simulink model "PFC_V10"  (R2016b)
settings: Solver=FixedStepDiscrete  StartTime=0.0  StopTime=0.1  FixedStep=1e-7  RelTol=1e-3
libraries: powerlib x15, simulink x1
settings Model: Creator=a037702  LastModifiedBy=a037702

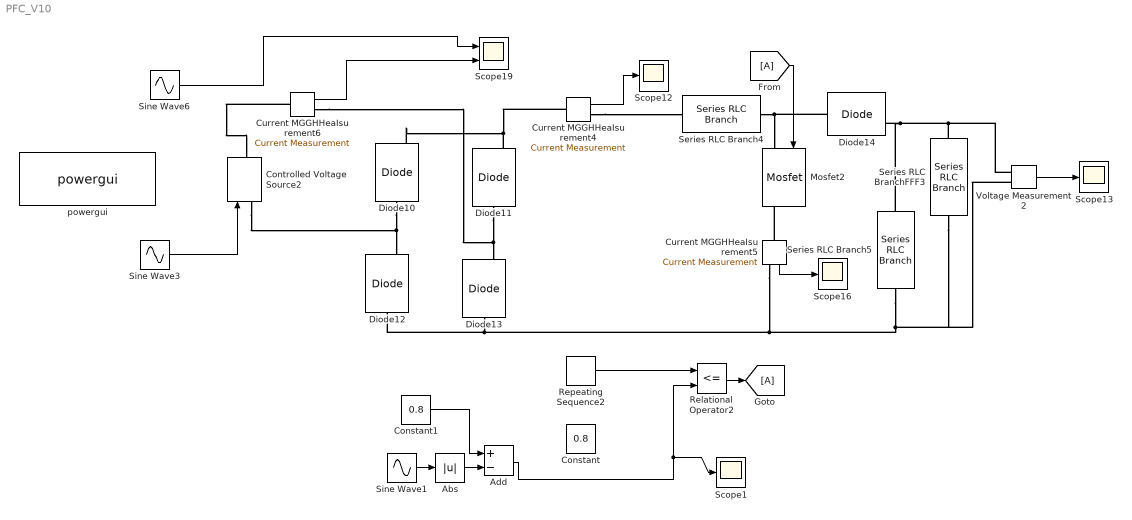
== system PFC_V10 ==
  Abs : Abs
  Add : Sum  Inputs=+-
  Constant : Constant  Value=0.8
  Constant1 : Constant  Value=0.8
  Controlled Voltage Source2 : powerlib/Electrical Sources/Controlled Voltage Source  Initialize=on  Source_Type=AC  Amplitude=0  Phase=0  Frequency=0  Measurements=None
  Current MGGHHeaIsurement4 : powerlib/Measurements/Current Measurement  PhasorSimulation=off  OutputType=Complex  PSBequivalent=0
  Current MGGHHeaIsurement5 : powerlib/Measurements/Current Measurement  PhasorSimulation=off  OutputType=Complex  PSBequivalent=0
  Current MGGHHeaIsurement6 : powerlib/Measurements/Current Measurement  PhasorSimulation=off  OutputType=Complex  PSBequivalent=0
  Diode{10..14} (5 alike) : powerlib/Power Electronics/Diode  Ron=0.001  Lon=0  Vf=0.8  IC=0  UseSnubber=off  Rs=500  Cs=250e-9  Measurements=on
  Mosfet2 : powerlib/Power Electronics/Mosfet  Ron=0.1  Lon=0  Rd=0.01  Vfd=0  IC=0  Rs=1e5  Cs=inf  Measurements=on
  Relational Operator2 : RelationalOperator  Operator=<=  OutDataTypeStr=boolean  RndMeth=Simplest
  Repeating Sequence2 : simulink/Sources/Repeating Sequence  rep_seq_t=[0 10e-6]  rep_seq_y=[0 1]
  Scope{1,12..13,16} (4 alike) : Scope
  Scope19 : Scope  NumInputPorts=2
  Series RLC Branch4 : powerlib/Elements/Series RLC Branch  LConnTagsString=__new0  RConnTagsString=__new0  BranchType=L  Resistance=1  Inductance=500e-6  SetiL0=on  InitialCurrent=0  Capacitance=1e-6  Setx0=off  InitialVoltage=0  Measurements=Branch current
  Series RLC Branch5 : powerlib/Elements/Series RLC Branch  LConnTagsString=__new0  RConnTagsString=__new0  BranchType=R  Resistance=100  Inductance=500e-6  SetiL0=on  InitialCurrent=0  Capacitance=100e-6  Setx0=on  InitialVoltage=0  Measurements=Branch current
  Series RLC BranchFFF3 : powerlib/Elements/Series RLC Branch  LConnTagsString=__new0  RConnTagsString=__new0  BranchType=C  Resistance=1  Inductance=500e-6  SetiL0=on  InitialCurrent=0  Capacitance=100e-6  Setx0=on  InitialVoltage=0  Measurements=Branch current
  Sine Wave1 : Sin  Amplitude=0.3  Frequency=2*pi*50  SampleTime=0
  Sine Wave3 : Sin  Amplitude=320  Frequency=2*pi*50  SampleTime=0
  Sine Wave6 : Sin  Amplitude=20  Frequency=2*pi*50  SampleTime=0
  Voltage Measurement2 : powerlib/Measurements/Voltage Measurement  PhasorSimulation=off  OutputType=Complex  PSBequivalent=0
  powergui : powerlib/powergui  Priority=1  SimulationMode=Discrete  SolverType=Tustin/Backward Euler (TBE)  SampleTime=.1e-6  frequency=60  SPID=off  DisableSnubberDevices=off  DisableRonSwitches=off  DisableVfSwitches=off  SwTol=0  DisplayEquations=off  Interpol=off  ExternalGateDelay=off  methode=off  Ts=10  FunctionMessages=off  echomessages=off  HookPort=off  EnableUseOfTLC=off  x0status=blocks  frequencyindice=0  Pbase=100e6  ErrMax=1e-4  Iterations=50  UnitsV=kV  UnitsW=MW  buscounter=0  RestoreLinks=warning  ResistiveCurrentMeasurement=off  Frange=[0:2:500]  Ylog=off  Xlog=on  ShowGrid=off  save=off  variable=ZData  structure=0  ZoomFFT=off  StartTime=0.0  cycles=1  DisplayStyle=1  fundamental=60  FreqAxis=off  MaxFrequency=1000  frequencyindicesteady=1  RmsSteady=1  display=off
  wires:
  Sine Wave3/1 -> Controlled Voltage Source2/1
  Current MGGHHeaIsurement4/1 -> Scope12/1
  Voltage Measurement2/1 -> Scope13/1
  Current MGGHHeaIsurement5/1 -> Scope16/1
  Repeating Sequence2/1 -> Relational Operator2/1
  Current MGGHHeaIsurement6/1 -> Scope19/2
  Sine Wave6/1 -> Scope19/1
  Add/1 -> Scope1/1, Relational Operator2/2
  Relational Operator2/1 -> [A]
  [A] -> Mosfet2/1
  Sine Wave1/1 -> Abs/1
  Abs/1 -> Add/2
  Constant1/1 -> Add/1
  connections:
  Diode11/RConn1 -- Diode10/RConn1 -- Current MGGHHeaIsurement4/LConn1
  Diode11/LConn1 -- Current MGGHHeaIsurement6/RConn1 -- Diode13/RConn1
  Diode10/LConn1 -- Controlled Voltage Source2/LConn1 -- Diode12/RConn1
  Diode13/LConn1 -- Series RLC Branch5/RConn1 -- Voltage Measurement2/LConn2 -- Series RLC BranchFFF3/RConn1 -- Current MGGHHeaIsurement5/RConn1 -- Diode12/LConn1
  Series RLC Branch4/RConn1 -- Diode14/LConn1 -- Mosfet2/LConn1
  Series RLC BranchFFF3/LConn1 -- Voltage Measurement2/LConn1 -- Series RLC Branch5/LConn1 -- Diode14/RConn1
  Current MGGHHeaIsurement4/RConn1 -- Series RLC Branch4/LConn1
  Current MGGHHeaIsurement5/LConn1 -- Mosfet2/RConn1
  Current MGGHHeaIsurement6/LConn1 -- Controlled Voltage Source2/RConn1
